simulink model "full_vehicle_sim"  (R2025b)
settings: Solver=VariableStepAuto  StartTime=0.0  StopTime=5  RelTol=1e-3
libraries: SimscapeFluids_lib x9, fl_lib x7, nesl_utility x5
(part 3 of 3)

== matlab function full_vehicle_sim/Vehicle Sim/Fuel Tank/MATLAB Function ==
  data: F_cmd input; u_fuel output
function u_fuel = fuel_controller(F_cmd)
% Input:
%   F_cmd [N]
%
% Output:
%   u_fuel [-]

    % ===== HARDCODED PARAMETERS =====
    MR_cmd = 2.5;
    Cf_cmd = 1.5;
    cstar_cmd = 1500;
    mdot_fuel_max = 0.5;

    % ===== TOTAL MDOT =====
    mdot_total_cmd = F_cmd / (Cf_cmd * cstar_cmd);

    % ===== SPLIT =====
    mdot_fuel_cmd = mdot_total_cmd / (1 + MR_cmd);

    % ===== VALVE SIGNAL =====
    u_fuel = mdot_fuel_cmd / mdot_fuel_max;

end

== matlab function full_vehicle_sim/Vehicle Sim/OX Tank/MATLAB Function ==
  data: F_cmd input; u_lox output
function u_lox = lox_controller(F_cmd)
% Input:
%   F_cmd [N]
%
% Output:
%   u_lox [-]

    % ===== HARDCODED PARAMETERS =====
    MR_cmd = 2.5;
    Cf_cmd = 1.5;
    cstar_cmd = 1500;
    mdot_lox_max = 1.0;

    % ===== TOTAL MDOT =====
    mdot_total_cmd = F_cmd / (Cf_cmd * cstar_cmd);

    % ===== SPLIT =====
    mdot_fuel_cmd = mdot_total_cmd / (1 + MR_cmd);
    mdot_lox_cmd  = MR_cmd * mdot_fuel_cmd;

    % ===== VALVE SIGNAL =====
    u_lox = mdot_lox_cmd / mdot_lox_max;

end

== matlab function full_vehicle_sim/Vehicle Sim/MATLAB Function ==
  data: mdot_ox input; F_actual output; mdot_fuel input; Pc output; MR_actual output; mdot_total output; cstar_eff output
function [F_actual, Pc, MR_actual, mdot_total, cstar_eff] = engine_model_actual_mdot(mdot_ox, mdot_fuel)
% Engine model using ACTUAL delivered mass flow rates
%
% Inputs:
%   mdot_ox   - actual oxidizer mass flow rate [kg/s]
%   mdot_fuel - actual fuel mass flow rate [kg/s]
%
% Outputs:
%   F_actual   - actual thrust [N]
%   Pc         - chamber pressure [Pa]
%   MR_actual  - actual mixture ratio [-]
%   mdot_total - total mass flow rate [kg/s]
%   cstar_eff  - effective characteristic velocity [m/s]

    % ===== PARAMETERS =====
    At = 1.0e-4;          % throat area [m^2]
    eta_cstar = 0.95;     % c* efficiency [-]
    cstar_ideal = 1550;   % ideal c* [m/s]
    Cf = 1.5;             % thrust coefficient [-]

    % ===== TOTAL FLOW =====
    mdot_total = mdot_ox + mdot_fuel;

    % ===== MIXTURE RATIO =====
    if mdot_fuel > 1e-8
        MR_actual = mdot_ox / mdot_fuel;
    else
        MR_actual = 0;
    end

    % ===== EFFECTIVE c* =====
    cstar_eff = eta_cstar * cstar_ideal;

    % ===== CHAMBER PRESSURE =====
    Pc = (mdot_total * cstar_eff) / At;

    % ===== ACTUAL THRUST =====
    F_actual = Cf * Pc * At;

    % same as:
    % F_actual = Cf * mdot_total * cstar_eff;

end

== matlab function full_vehicle_sim/Vehicle Sim/OX Side Tanks/OBB Control ==
  data: OTPT_A input; OBB_A output
function OBB_A  = fcn(OTPT_A)

if OTPT_A < 500
    OBB_A = 1;
else
    OBB_A = 0;
end

end

== matlab function full_vehicle_sim/Vehicle Sim/Fuel Side Tanks/FBB Control ==
  data: FTPT_A input; FBB_A output
function FBB_A  = fcn(FTPT_A)

if FTPT_A < 500
    FBB_A = 1;
else
    FBB_A = 0;
end

end
